simulink model "SMC"  (R2023a)
settings: Solver=FixedStepAuto  StartTime=0.0  StopTime=inf  RelTol=1e-3
undefined symbols (not defined in the file or in its folder): angular, linear
libraries: ros2lib x13

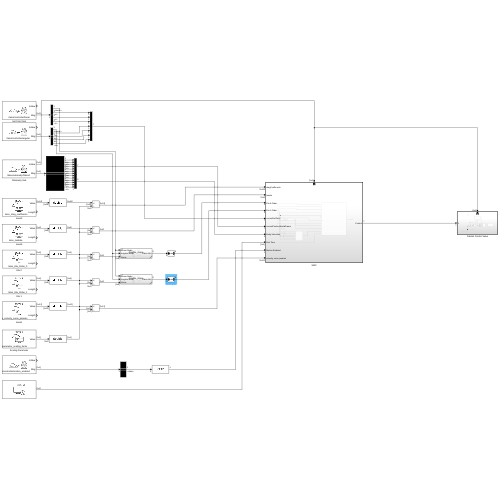
[thumbnail: Simulink's stored preview of the top-level diagram]
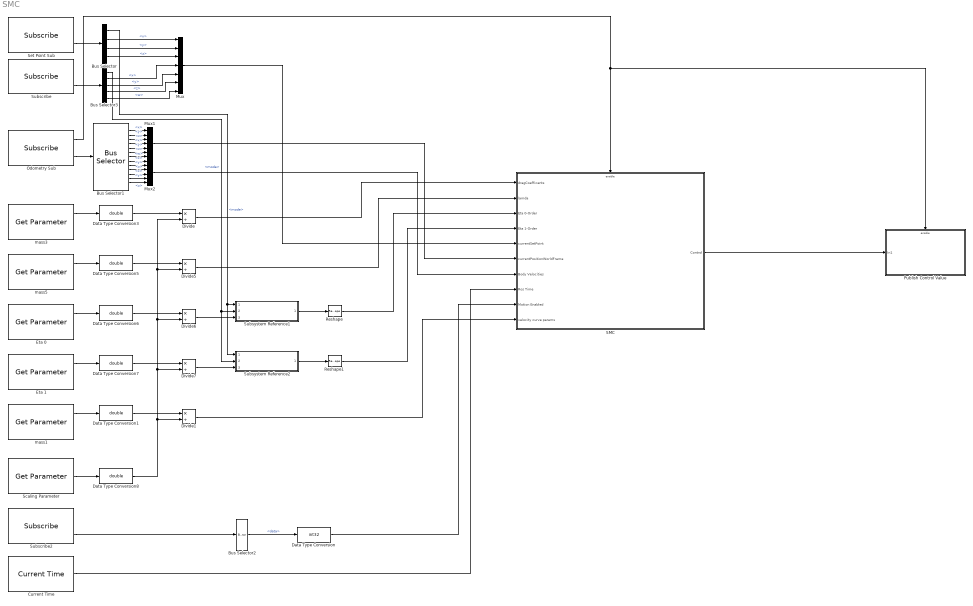
== system SMC ==
  Bus Selector : BusSelector  OutputSignals=mode,setpoint_vect.x,setpoint_vect.y,setpoint_vect.z
  Bus Selector1 : BusSelector  OutputSignals=pose.pose.position.x,pose.pose.position.y,pose.pose.position.z,pose.pose.orientation.x,pose.pose.orientation.y,pose.pose.orientation.z,pose.pose.orientation.w,twist.twist.linear.x,twist.twist.linear.y,twist.twist.linear.z,twist.twist.angular.x,twist.twist.angular.y,twist.twist.angular.z
  Bus Selector2 : BusSelector  OutputSignals=data
  Bus Selector3 : BusSelector  OutputSignals=mode,setpoint_quat.x,setpoint_quat.y,setpoint_quat.z,setpoint_quat.w
  Current Time : ros2lib/Current Time  OutputFormat=double  SampleTime=-1  ModelName=SMC
  Data Type Conversion : DataTypeConversion  OutDataTypeStr=int32  SaturateOnIntegerOverflow=off  RndMeth=Floor
  Data Type Conversion{1,3,5..8} (6 alike) : DataTypeConversion  OutDataTypeStr=double  SaturateOnIntegerOverflow=off  RndMeth=Floor
  Divide{,1,5..7} (5 alike) : Product  Inputs=*/
  Eta 0 : ros2lib/Get Parameter  ParameterName=talos_Eta_Order_0  ParameterType=int64[]  ParameterMaxArrayLength=6  ParameterInitialValue=0.0  SampleTime=-1  ModelName=SMC  BlockId=ParamGet_SMC_204
  Eta 1 : ros2lib/Get Parameter  ParameterName=talos_Eta_Order_1  ParameterType=int64[]  ParameterMaxArrayLength=6  ParameterInitialValue=0.0  SampleTime=-1  ModelName=SMC  BlockId=ParamGet_SMC_206
  Mux : Mux  Inputs=7
  Mux1 : Mux  Inputs=7
  Mux2 : Mux  Inputs=6
  Odometry Sub : ros2lib/Subscribe  topicSource=Specify your own  topic=/talos/odometry/filtered  messageType=nav_msgs/Odometry  sampleTime=0.01  QOSHistory=Keep last  QOSDepth=1  QOSReliability=Reliable  QOSDurability=Volatile
  Publish Control Value : Subsystem
  Reshape : Reshape  OutputDimensionality=Row vector (2-D)
  Reshape1 : Reshape  OutputDimensionality=Row vector (2-D)
  SMC : Subsystem
  Scaling Parameter : ros2lib/Get Parameter  ParameterName=parameter_scaling_factor  ParameterType=int64  ParameterMaxArrayLength=16  ParameterInitialValue=1000000  SampleTime=-1  ModelName=SMC  BlockId=ParamGet_SMC_208
  Set Point Sub : ros2lib/Subscribe  topicSource=Specify your own  topic=/talos/controller/linear  messageType=riptide_msgs2/ControllerCommand  sampleTime=0.01  QOSHistory=Keep last  QOSDepth=1  QOSReliability=Reliable  QOSDurability=Volatile
  Subscribe : ros2lib/Subscribe  topicSource=Specify your own  topic=/talos/controller/angular  messageType=riptide_msgs2/ControllerCommand  sampleTime=0.01  QOSHistory=Keep last  QOSDepth=1  QOSReliability=Reliable  QOSDurability=Volatile
  Subscribe2 : ros2lib/Subscribe  topicSource=Specify your own  topic=/talos/controller/motion_enabled  messageType=std_msgs/Bool  sampleTime=-1  QOSHistory=Keep last  QOSDepth=1  QOSReliability=Reliable  QOSDurability=Volatile
  Subsystem Reference1 : Subsystem  ReferencedSubsystem=Disable_Gains
  Subsystem Reference2 : Subsystem  ReferencedSubsystem=Disable_Gains
  mass1 : ros2lib/Get Parameter  ParameterName=talos_velocity_curve_params  ParameterType=int64[]  ParameterMaxArrayLength=12  ParameterInitialValue=[0,0,0,0,0,0,0,0,0,0,0,0]  SampleTime=-1  ModelName=SMC  BlockId=ParamGet_SMC_710
  mass3 : ros2lib/Get Parameter  ParameterName=talos_drag_coefficents  ParameterType=int64[]  ParameterMaxArrayLength=24  ParameterInitialValue=0.0  SampleTime=-1  ModelName=SMC  BlockId=ParamGet_SMC_197
  mass5 : ros2lib/Get Parameter  ParameterName=talos_lambda  ParameterType=int64[]  ParameterMaxArrayLength=6  ParameterInitialValue=0.0  SampleTime=-1  ModelName=SMC  BlockId=ParamGet_SMC_202
  wires:
  Mux/1 -> SMC/5(currentSetPoint)
  Odometry Sub/2 -> Bus Selector1/1
  Bus Selector1/1 -> Mux1/1  "<x>"
  Bus Selector1/2 -> Mux1/2  "<y>"
  Bus Selector1/3 -> Mux1/3  "<z>"
  Bus Selector1/4 -> Mux1/4  "<x>"
  Bus Selector1/5 -> Mux1/5  "<y>"
  Bus Selector1/6 -> Mux1/6  "<z>"
  Bus Selector1/7 -> Mux1/7  "<w>"
  Bus Selector1/8 -> Mux2/1  "<x>"
  Bus Selector1/9 -> Mux2/2  "<y>"
  Bus Selector1/10 -> Mux2/3  "<z>"
  Bus Selector1/11 -> Mux2/4  "<x>"
  Bus Selector1/12 -> Mux2/5  "<y>"
  Bus Selector1/13 -> Mux2/6  "<z>"
  Mux1/1 -> SMC/6(currentPositionWorldFrame)
  Mux2/1 -> SMC/7(Body Velocities)
  mass3/1 -> Data Type Conversion3/1
  mass5/1 -> Data Type Conversion5/1
  Eta 0/1 -> Data Type Conversion6/1
  Eta 1/1 -> Data Type Conversion7/1
  Scaling Parameter/1 -> Data Type Conversion8/1
  Data Type Conversion3/1 -> Divide/1
  Data Type Conversion5/1 -> Divide5/1
  Data Type Conversion6/1 -> Divide6/1
  Data Type Conversion7/1 -> Divide7/1
  Data Type Conversion8/1 -> Divide1/2, Divide7/2, Divide6/2, Divide/2, Divide5/2
  Divide/1 -> SMC/1(dragCoefficents)
  SMC/1(Control) -> Publish Control Value/1(In1)
  Odometry Sub/1 -> Publish Control Value/Enable, SMC/Enable
  Current Time/1 -> SMC/8(Ros Time)
  Subscribe2/2 -> Bus Selector2/1
  Bus Selector2/1 -> Data Type Conversion/1  "<data>"
  Data Type Conversion/1 -> SMC/9(Motion Enabled)
  mass1/1 -> Data Type Conversion1/1
  Data Type Conversion1/1 -> Divide1/1
  Divide1/1 -> SMC/10(velocity curve params)
  Set Point Sub/2 -> Bus Selector/1
  Bus Selector/2 -> Mux/1  "<x>"
  Bus Selector/3 -> Mux/2  "<y>"
  Bus Selector/4 -> Mux/3  "<z>"
  Subscribe/2 -> Bus Selector3/1
  Bus Selector3/2 -> Mux/4  "<x>"
  Bus Selector3/3 -> Mux/5  "<y>"
  Bus Selector3/4 -> Mux/6  "<z>"
  Bus Selector3/5 -> Mux/7  "<w>"
  Divide5/1 -> SMC/2(lamda)
  Divide6/1 -> Subsystem Reference1/3
  Subsystem Reference1/1 -> Reshape/1
  Divide7/1 -> Subsystem Reference2/3
  Subsystem Reference2/1 -> Reshape1/1
  Bus Selector/1 -> Subsystem Reference1/1, Subsystem Reference2/1  "<mode>"
  Bus Selector3/1 -> Subsystem Reference1/2, Subsystem Reference2/2  "<mode>"
  Reshape/1 -> SMC/3(Eta 0-Order)
  Reshape1/1 -> SMC/4(Eta 1-Order)

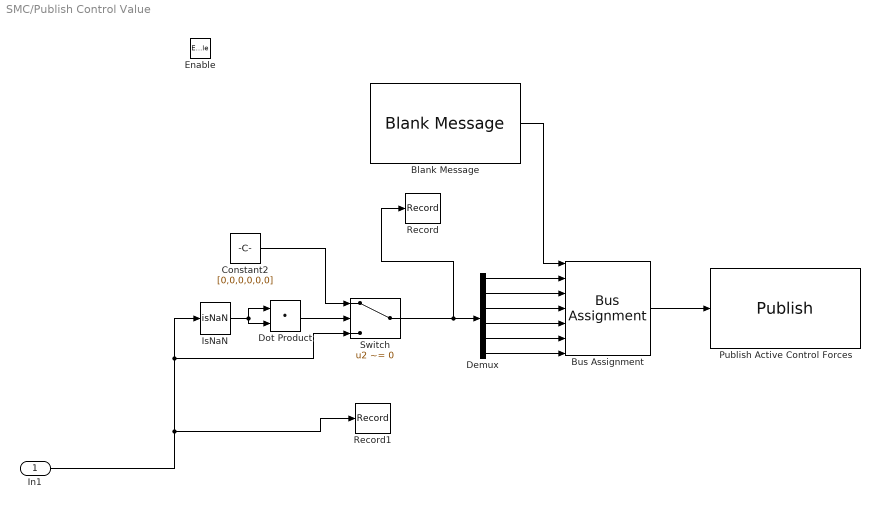
== system SMC/Publish Control Value ==
  In1 : Inport
  Enable : EnablePort
  Blank Message : ros2lib/Blank Message  messageClass=Message  entityType=geometry_msgs/Twist  messageType=geometry_msgs/Twist  SampleTime=inf
  Bus Assignment : BusAssignment  AssignedSignals=linear.x,linear.y,linear.z,angular.x,angular.y,angular.z
  Constant2 : Constant  Value=[0,0,0,0,0,0]
  Demux : Demux  Outputs=6
  Dot Product : DotProduct  OutDataTypeStr=Inherit: Inherit via internal rule
  IsNaN : RelationalOperator  Operator=isNaN  OutDataTypeStr=boolean  RndMeth=Simplest  InputSameDT=off
  Publish Active Control Forces : ros2lib/Publish  topicSource=Specify your own  topic=/talos/controller/active_body_force/smc  messageType=geometry_msgs/Twist  QOSHistory=Keep last  QOSDepth=1  QOSReliability=Reliable  QOSDurability=Volatile
  Record : Record  FileSettingsInternal="{\"entries\":[{\"content\":{\"excelSettings\":{\"content\":{},\"type\":\"Streamout.ExcelSettings\"}},\"type\":\"Streamout.FileSettingStorage\",\"uuid\":\"\"}],\"packageUris\":[\"http:\\/\\/schema.mathworks.com\\/mf0\\/streamout_blocks\\/R2020a\"],\"version\":\"1.0\"}"  Layout=[1 1]  SignalsInternal="{\"entries\":[{\"content\":{\"signals\":[{\"content\":{\"blockPath\":[],\"dimensions\":[6],\"domain\":\"\",\"hasChildren\":true,\"lineColor\":\"#77ac30\",\"port\":1,\"signalID\":4244,\"signalName\":\"Switch\"},\"type\":\"RecordBlkView.Signal\",\"uuid\":\"\"},{\"content\":{\"blockPath\":[],\"channel\":[1],\"dimensions\":[6],\"domain\":\"\",\"lineColor\":\"#77ac30\",\"parentID\":4244,\"port\":1,\"signalID\":4245,\"signalName\":\"Switch\"},\"type\":\"RecordBlkView.S ...(+1160 chars)"  VisualizationBindings="{\"sparklinesplugin\":{\"info\":[{\"bindingParametersList\":[],\"subplotID\":1}]}}"
  Record1 : Record  FileSettingsInternal="{\"entries\":[{\"content\":{\"excelSettings\":{\"content\":{},\"type\":\"Streamout.ExcelSettings\"}},\"type\":\"Streamout.FileSettingStorage\",\"uuid\":\"\"}],\"packageUris\":[\"http:\\/\\/schema.mathworks.com\\/mf0\\/streamout_blocks\\/R2020a\"],\"version\":\"1.0\"}"  Layout=[1 1]  SignalsInternal="{\"entries\":[{\"content\":{\"signals\":[{\"content\":{\"blockPath\":[],\"dimensions\":[6],\"domain\":\"\",\"hasChildren\":true,\"lineColor\":\"#a2142f\",\"port\":1,\"signalID\":4210,\"signalName\":\"In1\"},\"type\":\"RecordBlkView.Signal\",\"uuid\":\"\"},{\"content\":{\"blockPath\":[],\"channel\":[1],\"dimensions\":[6],\"domain\":\"\",\"lineColor\":\"#22b573\",\"parentID\":4210,\"plots\":[1],\"port\":1,\"signalID\":4211,\"signalName\":\"In1\"},\"type\":\"RecordBlk ...(+1199 chars)"  VisualizationBindings="{\"sparklinesplugin\":{\"info\":[{\"bindingParametersList\":[],\"subplotID\":1}]}}"
  Switch : Switch  Criteria=u2 ~= 0  SaturateOnIntegerOverflow=off  InputSameDT=off
  wires:
  Blank Message/1 -> Bus Assignment/1
  Switch/1 -> Record/1, Demux/1
  IsNaN/1 -> Dot Product/1, Dot Product/2
  Constant2/1 -> Switch/1
  Dot Product/1 -> Switch/2
  Demux/1 -> Bus Assignment/2
  Demux/2 -> Bus Assignment/3
  Demux/6 -> Bus Assignment/7
  Demux/3 -> Bus Assignment/4
  Demux/5 -> Bus Assignment/6
  In1/1 -> Record1/1, IsNaN/1, Switch/3
  Demux/4 -> Bus Assignment/5
  Bus Assignment/1 -> Publish Active Control Forces/1

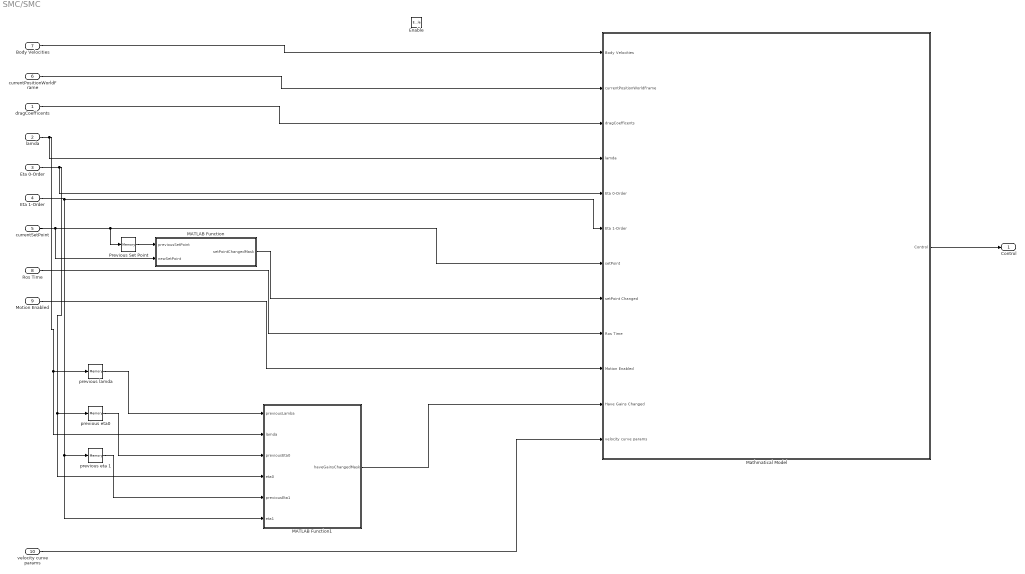
== system SMC/SMC ==
  dragCoefficents : Inport
  lamda : Inport  Port=2
  Eta 0-Order : Inport  Port=3
  Eta 1-Order : Inport  Port=4
  currentSetPoint : Inport  Port=5
  currentPositionWorldFrame : Inport  Port=6
  Body Velocities : Inport  Port=7
  Ros Time : Inport  Port=8
  Motion Enabled : Inport  Port=9
  velocity curve params : Inport  Port=10
  Enable : EnablePort
  MATLAB Function : MATLAB Function  TreatAsAtomicUnit=on
  MATLAB Function1 : MATLAB Function  TreatAsAtomicUnit=on
  Mathmatical Model : Subsystem
  Previous Set Point : Memory  InitialCondition=[0,0,0,0,0,0,0]  InheritSampleTime=on
  previous eta 1 : Memory  InheritSampleTime=on
  previous eta0 : Memory  InheritSampleTime=on
  previous lamda : Memory  InheritSampleTime=on
  Control : Outport
  wires:
  dragCoefficents/1 -> Mathmatical Model/3(dragCoefficents)
  Mathmatical Model/1(Control) -> Control/1
  currentSetPoint/1 -> MATLAB Function/2(newSetPoint), Previous Set Point/1, Mathmatical Model/7(setPoint)
  currentPositionWorldFrame/1 -> Mathmatical Model/2(currentPositionWorldFrame)
  Body Velocities/1 -> Mathmatical Model/1(Body Velocities)
  MATLAB Function/1(setPointChangedMask) -> Mathmatical Model/8(setPoint Changed)
  Previous Set Point/1 -> MATLAB Function/1(previousSetPoint)
  Ros Time/1 -> Mathmatical Model/9(Ros Time)
  Motion Enabled/1 -> Mathmatical Model/10(Motion Enabled)
  previous lamda/1 -> MATLAB Function1/1(previousLamba)
  previous eta0/1 -> MATLAB Function1/3(previousEta0)
  previous eta 1/1 -> MATLAB Function1/5(previousEta1)
  lamda/1 -> Mathmatical Model/4(lamda), MATLAB Function1/2(lamda), previous lamda/1
  Eta 0-Order/1 -> Mathmatical Model/5(Eta 0-Order), previous eta0/1, MATLAB Function1/4(eta0)
  Eta 1-Order/1 -> previous eta 1/1, MATLAB Function1/6(eta1), Mathmatical Model/6(Eta 1-Order)
  MATLAB Function1/1(haveGainsChangedMask) -> Mathmatical Model/11(Have Gains Changed)
  velocity curve params/1 -> Mathmatical Model/12(velocity curve params)

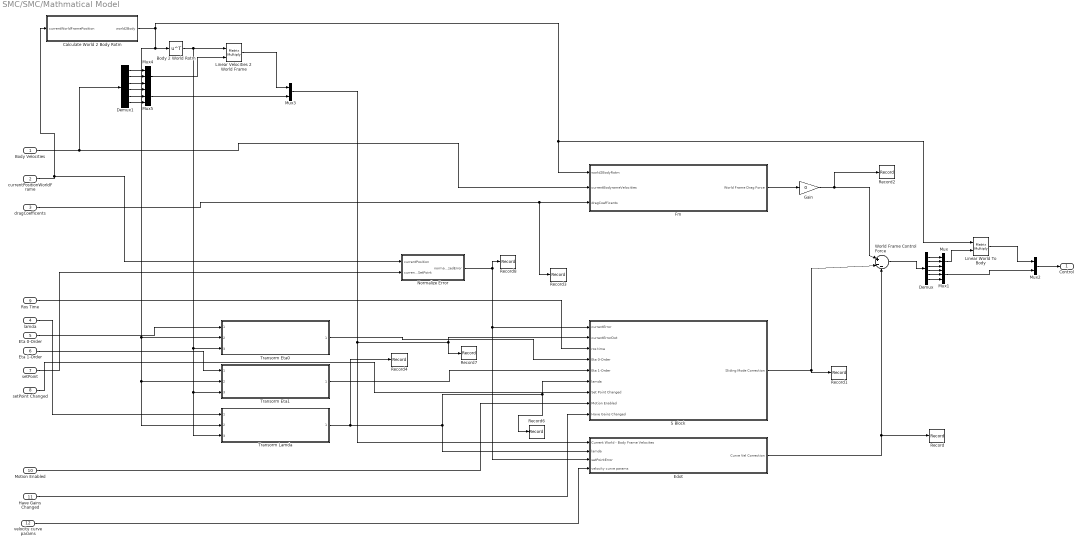
== system SMC/SMC/Mathmatical Model ==
  Body Velocities : Inport
  currentPositionWorldFrame : Inport  Port=2
  dragCoefficents : Inport  Port=3
  lamda : Inport  Port=4
  Eta 0-Order : Inport  Port=5
  Eta 1-Order : Inport  Port=6
  setPoint : Inport  Port=7
  setPoint Changed : Inport  Port=8
  Ros Time : Inport  Port=9
  Motion Enabled : Inport  Port=10
  Have Gains Changed : Inport  Port=11
  velocity curve params : Inport  Port=12
  Body 2 World Rotm : Math  Operator=transpose
  Calculate World 2 Body Rotm : MATLAB Function  TreatAsAtomicUnit=on
  Demux : Demux  Outputs=6
  Demux1 : Demux  Outputs=6
  Edot : Subsystem
  Fm : Subsystem
  Gain : Gain  Gain=0
  Linear Velocities 2 World Frame : Product  Multiplication=Matrix(*)
  Linear World To Body : Product  Multiplication=Matrix(*)
  Mux{,1,4..5} (4 alike) : Mux  Inputs=3
  Mux2 : Mux  Inputs=2
  Mux3 : Mux  Inputs=2
  Normalize Error : MATLAB Function  TreatAsAtomicUnit=on
  Record : Record  FileSettingsInternal="{\"entries\":[{\"content\":{\"excelSettings\":{\"content\":{},\"type\":\"Streamout.ExcelSettings\"}},\"type\":\"Streamout.FileSettingStorage\",\"uuid\":\"\"}],\"packageUris\":[\"http:\\/\\/schema.mathworks.com\\/mf0\\/streamout_blocks\\/R2020a\"],\"version\":\"1.0\"}"  Layout=[1 1]  SignalsInternal="{\"entries\":[{\"content\":{\"signals\":[{\"content\":{\"blockPath\":[],\"dimensions\":[6,1],\"domain\":\"\",\"hasChildren\":true,\"lineColor\":\"#ff13a6\",\"port\":1,\"signalID\":4045,\"signalName\":\"Edot\"},\"type\":\"RecordBlkView.Signal\",\"uuid\":\"\"},{\"content\":{\"blockPath\":[],\"channel\":[1,1],\"dimensions\":[6,1],\"domain\":\"\",\"lineColor\":\"#4dbeee\",\"parentID\":4045,\"port\":1,\"signalID\":4046,\"signalName\":\"Edot\"},\"type\":\"RecordBlkView ...(+1172 chars)"  VisualizationBindings="{\"sparklinesplugin\":{\"info\":[{\"bindingParametersList\":[],\"subplotID\":1}]}}"
  Record1 : Record  FileSettingsInternal="{\"entries\":[{\"content\":{\"excelSettings\":{\"content\":{},\"type\":\"Streamout.ExcelSettings\"}},\"type\":\"Streamout.FileSettingStorage\",\"uuid\":\"\"}],\"packageUris\":[\"http:\\/\\/schema.mathworks.com\\/mf0\\/streamout_blocks\\/R2020a\"],\"version\":\"1.0\"}"  Layout=[1 1]  SignalsInternal="{\"entries\":[{\"content\":{\"signals\":[{\"content\":{\"blockPath\":[],\"dimensions\":[6,1],\"domain\":\"\",\"hasChildren\":true,\"lineColor\":\"#22b573\",\"port\":1,\"signalID\":4227,\"signalName\":\"S Block\"},\"type\":\"RecordBlkView.Signal\",\"uuid\":\"\"},{\"content\":{\"blockPath\":[],\"channel\":[1,1],\"dimensions\":[6,1],\"domain\":\"\",\"lineColor\":\"#0072bd\",\"parentID\":4227,\"port\":1,\"signalID\":4228,\"signalName\":\"S Block\"},\"type\":\"RecordB ...(+1193 chars)"  VisualizationBindings="{\"sparklinesplugin\":{\"info\":[{\"bindingParametersList\":[],\"subplotID\":1}]}}"
  Record2 : Record  FileSettingsInternal="{\"entries\":[{\"content\":{\"excelSettings\":{\"content\":{},\"type\":\"Streamout.ExcelSettings\"}},\"type\":\"Streamout.FileSettingStorage\",\"uuid\":\"\"}],\"packageUris\":[\"http:\\/\\/schema.mathworks.com\\/mf0\\/streamout_blocks\\/R2020a\"],\"version\":\"1.0\"}"  Layout=[1 1]  SignalsInternal="{\"entries\":[{\"content\":{\"signals\":[{\"content\":{\"blockPath\":[],\"dimensions\":[6],\"domain\":\"\",\"hasChildren\":true,\"lineColor\":\"#d95319\",\"port\":1,\"signalID\":3994,\"signalName\":\"Gain\"},\"type\":\"RecordBlkView.Signal\",\"uuid\":\"\"},{\"content\":{\"blockPath\":[],\"channel\":[1],\"dimensions\":[6],\"domain\":\"\",\"lineColor\":\"#edb120\",\"parentID\":3994,\"plots\":[1],\"port\":1,\"signalID\":3995,\"signalName\":\"Gain\"},\"type\":\"RecordB ...(+1206 chars)"  VisualizationBindings="{\"sparklinesplugin\":{\"info\":[{\"bindingParametersList\":[],\"subplotID\":1}]}}"
  Record3 : Record  FileSettingsInternal="{\"entries\":[{\"content\":{\"excelSettings\":{\"content\":{},\"type\":\"Streamout.ExcelSettings\"}},\"type\":\"Streamout.FileSettingStorage\",\"uuid\":\"\"}],\"packageUris\":[\"http:\\/\\/schema.mathworks.com\\/mf0\\/streamout_blocks\\/R2020a\"],\"version\":\"1.0\"}"  Layout=[1 1]  SignalsInternal="{\"entries\":[{\"content\":{\"signals\":[{\"content\":{\"blockPath\":[],\"dimensions\":[1,24],\"domain\":\"\",\"hasChildren\":true,\"lineColor\":\"#7e2f8e\",\"port\":1,\"signalID\":3941,\"signalName\":\"dragCoefficents\"},\"type\":\"RecordBlkView.Signal\",\"uuid\":\"\"},{\"content\":{\"blockPath\":[],\"channel\":[1,1],\"dimensions\":[1,24],\"domain\":\"\",\"lineColor\":\"#77ac30\",\"parentID\":3941,\"plots\":[1],\"port\":1,\"signalID\":3942,\"signalName\":\"dra ...(+5141 chars)"  VisualizationBindings="{\"sparklinesplugin\":{\"info\":[{\"bindingParametersList\":[],\"subplotID\":1}]}}"
  Record4 : Record  FileSettingsInternal="{\"entries\":[{\"content\":{\"excelSettings\":{\"content\":{},\"type\":\"Streamout.ExcelSettings\"}},\"type\":\"Streamout.FileSettingStorage\",\"uuid\":\"\"}],\"packageUris\":[\"http:\\/\\/schema.mathworks.com\\/mf0\\/streamout_blocks\\/R2020a\"],\"version\":\"1.0\"}"  Layout=[1 1]  SignalsInternal="{\"entries\":[{\"content\":{\"signals\":[{\"content\":{\"blockPath\":[],\"dimensions\":[6],\"domain\":\"\",\"hasChildren\":true,\"lineColor\":\"#4dbeee\",\"port\":1,\"signalID\":3907,\"signalName\":\"Transorm Lamda\"},\"type\":\"RecordBlkView.Signal\",\"uuid\":\"\"},{\"content\":{\"blockPath\":[],\"channel\":[1],\"dimensions\":[6],\"domain\":\"\",\"lineColor\":\"#64d413\",\"parentID\":3907,\"plots\":[1],\"port\":1,\"signalID\":3908,\"signalName\":\"Transorm Lam ...(+1276 chars)"  VisualizationBindings="{\"sparklinesplugin\":{\"info\":[{\"bindingParametersList\":[],\"subplotID\":1}]}}"
  Record6 : Record  FileSettingsInternal="{\"entries\":[{\"content\":{\"excelSettings\":{\"content\":{},\"type\":\"Streamout.ExcelSettings\"}},\"type\":\"Streamout.FileSettingStorage\",\"uuid\":\"\"}],\"packageUris\":[\"http:\\/\\/schema.mathworks.com\\/mf0\\/streamout_blocks\\/R2020a\"],\"version\":\"1.0\"}"  Layout=[1 1]  SignalsInternal="{\"entries\":[{\"content\":{\"signals\":[{\"content\":{\"blockPath\":[],\"dimensions\":[6],\"domain\":\"\",\"hasChildren\":true,\"lineColor\":\"#139fff\",\"port\":1,\"signalID\":3924,\"signalName\":\"Transorm Lamda\"},\"type\":\"RecordBlkView.Signal\",\"uuid\":\"\"},{\"content\":{\"blockPath\":[],\"channel\":[1],\"dimensions\":[6],\"domain\":\"\",\"lineColor\":\"#64d413\",\"parentID\":3924,\"plots\":[1],\"port\":1,\"signalID\":3925,\"signalName\":\"Transorm Lam ...(+1240 chars)"  VisualizationBindings="{\"sparklinesplugin\":{\"info\":[{\"bindingParametersList\":[],\"subplotID\":1}]}}"
  Record7 : Record  FileSettingsInternal="{\"entries\":[{\"content\":{\"excelSettings\":{\"content\":{},\"type\":\"Streamout.ExcelSettings\"}},\"type\":\"Streamout.FileSettingStorage\",\"uuid\":\"\"}],\"packageUris\":[\"http:\\/\\/schema.mathworks.com\\/mf0\\/streamout_blocks\\/R2020a\"],\"version\":\"1.0\"}"  Layout=[1 1]  SignalsInternal="{\"entries\":[{\"content\":{\"signals\":[{\"content\":{\"blockPath\":[],\"dimensions\":[6],\"domain\":\"\",\"hasChildren\":true,\"lineColor\":\"#b746ff\",\"port\":1,\"signalID\":4011,\"signalName\":\"Mux3\"},\"type\":\"RecordBlkView.Signal\",\"uuid\":\"\"},{\"content\":{\"blockPath\":[],\"channel\":[1],\"dimensions\":[6],\"domain\":\"\",\"lineColor\":\"#edb120\",\"parentID\":4011,\"plots\":[1],\"port\":1,\"signalID\":4012,\"signalName\":\"Mux3\"},\"type\":\"RecordB ...(+1170 chars)"  VisualizationBindings="{\"sparklinesplugin\":{\"info\":[{\"bindingParametersList\":[],\"subplotID\":1}]}}"
  Record8 : Record  FileSettingsInternal="{\"entries\":[{\"content\":{\"excelSettings\":{\"content\":{},\"type\":\"Streamout.ExcelSettings\"}},\"type\":\"Streamout.FileSettingStorage\",\"uuid\":\"\"}],\"packageUris\":[\"http:\\/\\/schema.mathworks.com\\/mf0\\/streamout_blocks\\/R2020a\"],\"version\":\"1.0\"}"  Layout=[1 1]  SignalsInternal="{\"entries\":[{\"content\":{\"signals\":[{\"content\":{\"blockPath\":[],\"dimensions\":[1,6],\"domain\":\"\",\"hasChildren\":true,\"lineColor\":\"#ff13a6\",\"port\":1,\"signalID\":4028,\"signalName\":\"Normalize Error\"},\"type\":\"RecordBlkView.Signal\",\"uuid\":\"\"},{\"content\":{\"blockPath\":[],\"channel\":[1,1],\"dimensions\":[1,6],\"domain\":\"\",\"lineColor\":\"#a2142f\",\"parentID\":4028,\"plots\":[1],\"port\":1,\"signalID\":4029,\"signalName\":\"Norma ...(+1273 chars)"  VisualizationBindings="{\"sparklinesplugin\":{\"info\":[{\"bindingParametersList\":[],\"subplotID\":1}]}}"
  S Block : Subsystem
  Transorm Eta0 : Subsystem  ReferencedSubsystem=Tranfsform_Linear_Gains_To_World
  Transorm Eta1 : Subsystem  ReferencedSubsystem=Tranfsform_Linear_Gains_To_World
  Transorm Lamda : Subsystem  ReferencedSubsystem=Tranfsform_Linear_Gains_To_World
  World Frame Control Force : Sum  Inputs=|+--
  Control : Outport
  wires:
  Body Velocities/1 -> Fm/2(currentBodyrameVelocities), Demux1/1
  currentPositionWorldFrame/1 -> Normalize Error/1(currentPosition), Calculate World 2 Body Rotm/1(currentWorldFramePosition)
  S Block/1("Sliding Mode Correction ") -> World Frame Control Force/2, Record1/1
  World Frame Control Force/1 -> Demux/1
  Demux/1 -> Mux/1
  Demux/2 -> Mux/2
  Demux/3 -> Mux/3
  Demux/6 -> Mux1/3
  Demux/5 -> Mux1/2
  Demux/4 -> Mux1/1
  Mux/1 -> Linear World To Body/2
  Linear World To Body/1 -> Mux2/1
  Mux1/1 -> Mux2/2
  Mux2/1 -> Control/1
  Calculate World 2 Body Rotm/1(world2Body) -> Body 2 World Rotm/1, Transorm Eta0/2, Transorm Eta1/2, Transorm Lamda/2, Linear World To Body/1, Fm/1(world2BodyRotm)
  dragCoefficents/1 -> Record3/1, Fm/3(dragCoefficents)
  Linear Velocities 2 World Frame/1 -> Mux3/1
  Mux4/1 -> Linear Velocities 2 World Frame/2
  Demux1/2 -> Mux4/2
  Demux1/1 -> Mux4/1
  Demux1/3 -> Mux4/3
  Demux1/5 -> Mux5/2
  Demux1/4 -> Mux5/1
  Demux1/6 -> Mux5/3
  Fm/1(World Frame Drag Force) -> Gain/1
  Mux5/1 -> Mux3/2
  Transorm Lamda/1 -> Record4/1, Record6/1, S Block/6(lamda), Edot/2(lamda)
  Transorm Eta1/1 -> S Block/5(Eta 1-Order)
  lamda/1 -> Transorm Lamda/1
  Eta 0-Order/1 -> Transorm Eta0/1
  Mux3/1 -> Record7/1, S Block/2(currentErrorDot), Edot/1(Current World - Body Frame Velocites)
  setPoint Changed/1 -> S Block/7(Set Point Changed)
  Ros Time/1 -> S Block/3(ros time)
  Normalize Error/1(normalizedError) -> Record8/1, Edot/3(setPointError), S Block/1(currentError)
  setPoint/1 -> Normalize Error/2(currentSetPoint)
  Eta 1-Order/1 -> Transorm Eta1/1
  Gain/1 -> Record2/1, World Frame Control Force/1
  Edot/1(Curve Vel Correction) -> Record/1, World Frame Control Force/3
  Body 2 World Rotm/1 -> Transorm Eta0/3, Transorm Eta1/3, Transorm Lamda/3, Linear Velocities 2 World Frame/1
  Transorm Eta0/1 -> S Block/4(Eta 0-Order)
  Motion Enabled/1 -> S Block/8(Motion Enabled)
  Have Gains Changed/1 -> S Block/9(Have Gains Changed)
  velocity curve params/1 -> Edot/4(velocity curve params)

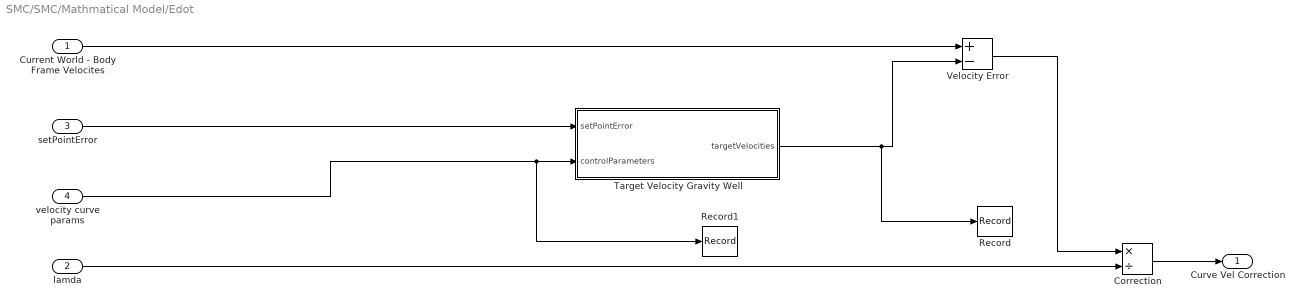
== system SMC/SMC/Mathmatical Model/Edot ==
  Current World - Body Frame Velocites : Inport
  lamda : Inport  Port=2
  setPointError : Inport  Port=3
  velocity curve params : Inport  Port=4
  Correction : Product  Inputs=*/
  Record : Record  FileSettingsInternal="{\"entries\":[{\"content\":{\"excelSettings\":{\"content\":{},\"type\":\"Streamout.ExcelSettings\"}},\"type\":\"Streamout.FileSettingStorage\",\"uuid\":\"\"}],\"packageUris\":[\"http:\\/\\/schema.mathworks.com\\/mf0\\/streamout_blocks\\/R2020a\"],\"version\":\"1.0\"}"  Layout=[1 1]  SignalsInternal="{\"entries\":[{\"content\":{\"signals\":[{\"content\":{\"blockPath\":[],\"dimensions\":[6,1],\"domain\":\"\",\"hasChildren\":true,\"lineColor\":\"#22b573\",\"port\":1,\"signalID\":4153,\"signalName\":\"Target Velocity Gravity Well\"},\"type\":\"RecordBlkView.Signal\",\"uuid\":\"\"},{\"content\":{\"blockPath\":[],\"channel\":[1,1],\"dimensions\":[6,1],\"domain\":\"\",\"lineColor\":\"#d95319\",\"parentID\":4153,\"plots\":[1],\"port\":1,\"signalID\":4154,\"signa ...(+1340 chars)"  VisualizationBindings="{\"sparklinesplugin\":{\"info\":[{\"bindingParametersList\":[],\"subplotID\":1}]}}"
  Record1 : Record  FileSettingsInternal="{\"entries\":[{\"content\":{\"excelSettings\":{\"content\":{},\"type\":\"Streamout.ExcelSettings\"}},\"type\":\"Streamout.FileSettingStorage\",\"uuid\":\"\"}],\"packageUris\":[\"http:\\/\\/schema.mathworks.com\\/mf0\\/streamout_blocks\\/R2020a\"],\"version\":\"1.0\"}"  Layout=[1 1]  SignalsInternal="{\"entries\":[{\"content\":{\"signals\":[{\"content\":{\"blockPath\":[],\"dimensions\":[1,12],\"domain\":\"\",\"hasChildren\":true,\"lineColor\":\"#d95319\",\"port\":1,\"signalID\":4170,\"signalName\":\"velocity curve params\"},\"type\":\"RecordBlkView.Signal\",\"uuid\":\"\"},{\"content\":{\"blockPath\":[],\"channel\":[1,1],\"dimensions\":[1,12],\"domain\":\"\",\"lineColor\":\"#edb120\",\"parentID\":4170,\"plots\":[1],\"port\":1,\"signalID\":4171,\"signalName ...(+2639 chars)"  VisualizationBindings="{\"sparklinesplugin\":{\"info\":[{\"bindingParametersList\":[],\"subplotID\":1}]}}"
  Target Velocity Gravity Well : MATLAB Function  TreatAsAtomicUnit=on
  Velocity Error : Sum  Inputs=+-
  Curve Vel Correction : Outport
  wires:
  Correction/1 -> Curve Vel Correction/1
  lamda/1 -> Correction/2
  Current World - Body Frame Velocites/1 -> Velocity Error/1
  Velocity Error/1 -> Correction/1
  setPointError/1 -> Target Velocity Gravity Well/1(setPointError)
  Target Velocity Gravity Well/1(targetVelocities) -> Record/1, Velocity Error/2
  velocity curve params/1 -> Record1/1, Target Velocity Gravity Well/2(controlParameters)

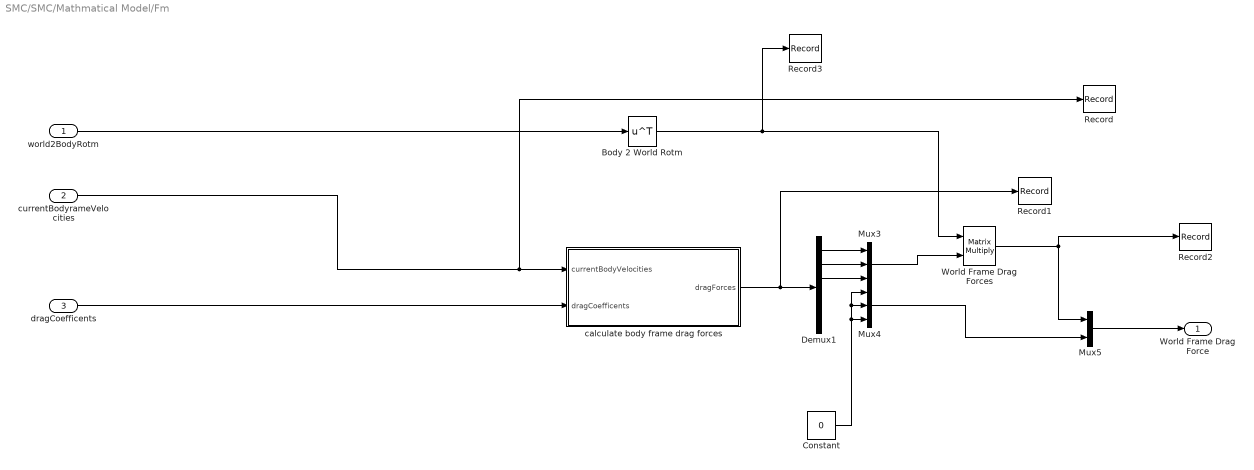
== system SMC/SMC/Mathmatical Model/Fm ==
  world2BodyRotm : Inport
  currentBodyrameVelocities : Inport  Port=2
  dragCoefficents : Inport  Port=3
  Body 2 World Rotm : Math  Operator=transpose
  Constant : Constant  Value=0
  Demux1 : Demux  Outputs=6
  Mux3 : Mux  Inputs=3
  Mux4 : Mux  Inputs=3
  Mux5 : Mux  Inputs=2
  Record : Record  FileSettingsInternal="{\"entries\":[{\"content\":{\"excelSettings\":{\"content\":{},\"type\":\"Streamout.ExcelSettings\"}},\"type\":\"Streamout.FileSettingStorage\",\"uuid\":\"\"}],\"packageUris\":[\"http:\\/\\/schema.mathworks.com\\/mf0\\/streamout_blocks\\/R2020a\"],\"version\":\"1.0\"}"  Layout=[1 1]  SignalsInternal="{\"entries\":[{\"content\":{\"signals\":[{\"content\":{\"blockPath\":[],\"dimensions\":[6],\"domain\":\"\",\"hasChildren\":true,\"lineColor\":\"#7e2f8e\",\"port\":1,\"signalID\":4119,\"signalName\":\"currentBodyrameVelocities\"},\"type\":\"RecordBlkView.Signal\",\"uuid\":\"\"},{\"content\":{\"blockPath\":[],\"channel\":[1],\"dimensions\":[6],\"domain\":\"\",\"lineColor\":\"#b746ff\",\"parentID\":4119,\"plots\":[1],\"port\":1,\"signalID\":4120,\"signalName\":\"c ...(+1341 chars)"  VisualizationBindings="{\"sparklinesplugin\":{\"info\":[{\"bindingParametersList\":[],\"subplotID\":1}]}}"
  Record1 : Record  FileSettingsInternal="{\"entries\":[{\"content\":{\"excelSettings\":{\"content\":{},\"type\":\"Streamout.ExcelSettings\"}},\"type\":\"Streamout.FileSettingStorage\",\"uuid\":\"\"}],\"packageUris\":[\"http:\\/\\/schema.mathworks.com\\/mf0\\/streamout_blocks\\/R2020a\"],\"version\":\"1.0\"}"  Layout=[1 1]  SignalsInternal="{\"entries\":[{\"content\":{\"signals\":[{\"content\":{\"blockPath\":[],\"dimensions\":[6,1],\"domain\":\"\",\"hasChildren\":true,\"lineColor\":\"#4dbeee\",\"port\":1,\"signalID\":4085,\"signalName\":\"calculate body frame drag forces\"},\"type\":\"RecordBlkView.Signal\",\"uuid\":\"\"},{\"content\":{\"blockPath\":[],\"channel\":[1,1],\"dimensions\":[6,1],\"domain\":\"\",\"lineColor\":\"#139fff\",\"parentID\":4085,\"plots\":[1],\"port\":1,\"signalID\":4086,\"s ...(+1428 chars)"  VisualizationBindings="{\"sparklinesplugin\":{\"info\":[{\"bindingParametersList\":[],\"subplotID\":1}]}}"
  Record2 : Record  FileSettingsInternal="{\"entries\":[{\"content\":{\"excelSettings\":{\"content\":{},\"type\":\"Streamout.ExcelSettings\"}},\"type\":\"Streamout.FileSettingStorage\",\"uuid\":\"\"}],\"packageUris\":[\"http:\\/\\/schema.mathworks.com\\/mf0\\/streamout_blocks\\/R2020a\"],\"version\":\"1.0\"}"  SignalsInternal="{\"entries\":[{\"content\":{\"signals\":[{\"content\":{\"blockPath\":[],\"dimensions\":[3],\"domain\":\"\",\"hasChildren\":true,\"lineColor\":\"#139fff\",\"port\":1,\"signalID\":4199,\"signalName\":\"World Frame Drag Forces\"},\"type\":\"RecordBlkView.Signal\",\"uuid\":\"\"},{\"content\":{\"blockPath\":[],\"channel\":[1],\"dimensions\":[3],\"domain\":\"\",\"lineColor\":\"#b746ff\",\"parentID\":4199,\"plots\":[1],\"port\":1,\"signalID\":4200,\"signalName\":\"Wor ...(+661 chars)"  VisualizationBindings="{\"sparklinesplugin\":{\"info\":[{\"bindingParametersList\":[],\"subplotID\":1}]}}"
  Record3 : Record  FileSettingsInternal="{\"entries\":[{\"content\":{\"excelSettings\":{\"content\":{},\"type\":\"Streamout.ExcelSettings\"}},\"type\":\"Streamout.FileSettingStorage\",\"uuid\":\"\"}],\"packageUris\":[\"http:\\/\\/schema.mathworks.com\\/mf0\\/streamout_blocks\\/R2020a\"],\"version\":\"1.0\"}"  Layout=[1 1]  SignalsInternal="{\"entries\":[{\"content\":{\"signals\":[{\"content\":{\"blockPath\":[],\"dimensions\":[3,3],\"domain\":\"\",\"hasChildren\":true,\"lineColor\":\"#b746ff\",\"port\":1,\"signalID\":4062,\"signalName\":\"Body 2 World Rotm\"},\"type\":\"RecordBlkView.Signal\",\"uuid\":\"\"},{\"content\":{\"blockPath\":[],\"channel\":[1,1],\"dimensions\":[3,3],\"domain\":\"\",\"lineColor\":\"#a2142f\",\"parentID\":4062,\"plots\":[1],\"port\":1,\"signalID\":4063,\"signalName\":\"Bod ...(+1995 chars)"  VisualizationBindings="{\"sparklinesplugin\":{\"info\":[{\"bindingParametersList\":[],\"subplotID\":1}]}}"
  World Frame Drag Forces : Product  Multiplication=Matrix(*)
  calculate body frame drag forces : MATLAB Function  TreatAsAtomicUnit=on
  World Frame Drag Force : Outport
  wires:
  World Frame Drag Forces/1 -> Mux5/1, Record2/1
  Demux1/1 -> Mux3/1
  Mux3/1 -> World Frame Drag Forces/2
  Demux1/3 -> Mux3/3
  Mux5/1 -> World Frame Drag Force/1
  Demux1/2 -> Mux3/2
  currentBodyrameVelocities/1 -> Record/1, calculate body frame drag forces/1(currentBodyVelocities)
  dragCoefficents/1 -> calculate body frame drag forces/2(dragCoefficents)
  world2BodyRotm/1 -> Body 2 World Rotm/1
  Body 2 World Rotm/1 -> Record3/1, World Frame Drag Forces/1
  calculate body frame drag forces/1(dragForces) -> Record1/1, Demux1/1
  Mux4/1 -> Mux5/2
  Constant/1 -> Mux4/3, Mux4/2, Mux4/1

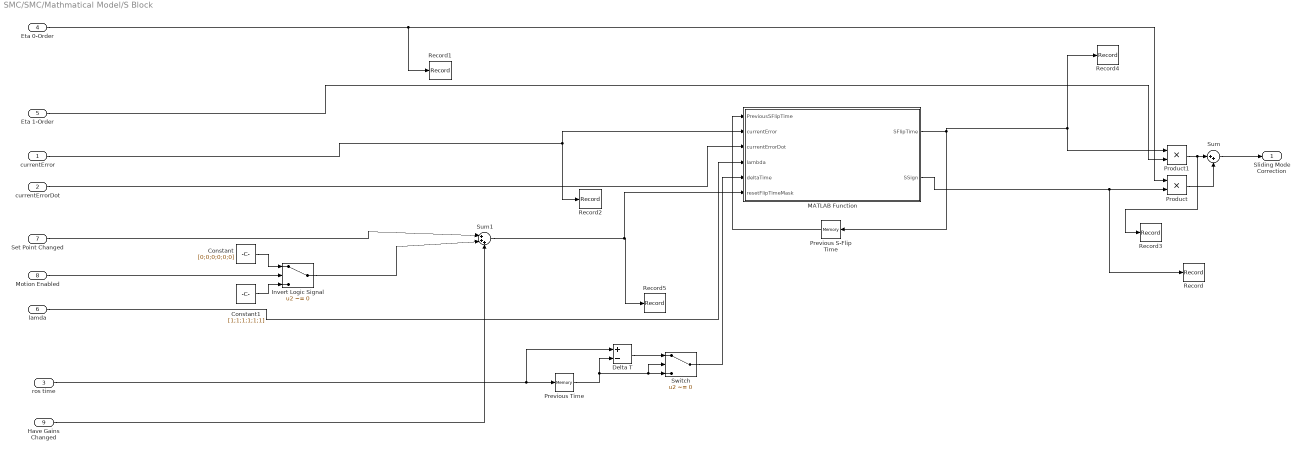
== system SMC/SMC/Mathmatical Model/S Block ==
  currentError : Inport
  currentErrorDot : Inport  Port=2
  ros time : Inport  Port=3
  Eta 0-Order : Inport  Port=4
  Eta 1-Order : Inport  Port=5
  lamda : Inport  Port=6
  Set Point Changed : Inport  Port=7
  Motion Enabled : Inport  Port=8
  Have Gains Changed : Inport  Port=9
  Constant : Constant  Value=[0;0;0;0;0;0]
  Constant1 : Constant  Value=[1;1;1;1;1;1]
  Delta T : Sum  Inputs=+-
  Invert Logic Signal : Switch  Criteria=u2 ~= 0  SaturateOnIntegerOverflow=off  InputSameDT=off
  MATLAB Function : MATLAB Function  TreatAsAtomicUnit=on
  Previous S-Flip Time : Memory  InitialCondition=[0;0;0;0;0;0]  InheritSampleTime=on
  Previous Time : Memory  InheritSampleTime=on
  Product : Product
  Product1 : Product
  Record : Record  FileSettingsInternal="{\"entries\":[{\"content\":{\"excelSettings\":{\"content\":{},\"type\":\"Streamout.ExcelSettings\"}},\"type\":\"Streamout.FileSettingStorage\",\"uuid\":\"\"}],\"packageUris\":[\"http:\\/\\/schema.mathworks.com\\/mf0\\/streamout_blocks\\/R2020a\"],\"version\":\"1.0\"}"  Layout=[1 1]  SignalsInternal="{\"entries\":[{\"content\":{\"signals\":[{\"content\":{\"blockPath\":[],\"dimensions\":[6,1],\"domain\":\"\",\"hasChildren\":true,\"lineColor\":\"#ff13a6\",\"port\":1,\"signalID\":3890,\"signalName\":\"MATLAB Function:2\"},\"type\":\"RecordBlkView.Signal\",\"uuid\":\"\"},{\"content\":{\"blockPath\":[],\"channel\":[1,1],\"dimensions\":[6,1],\"domain\":\"\",\"lineColor\":\"#77ac30\",\"parentID\":3890,\"plots\":[1],\"port\":1,\"signalID\":3891,\"signalName\":\"MAT ...(+1287 chars)"  VisualizationBindings="{\"sparklinesplugin\":{\"info\":[{\"bindingParametersList\":[],\"subplotID\":1}]}}"
  Record1 : Record  FileSettingsInternal="{\"entries\":[{\"content\":{\"excelSettings\":{\"content\":{},\"type\":\"Streamout.ExcelSettings\"}},\"type\":\"Streamout.FileSettingStorage\",\"uuid\":\"\"}],\"packageUris\":[\"http:\\/\\/schema.mathworks.com\\/mf0\\/streamout_blocks\\/R2020a\"],\"version\":\"1.0\"}"  Layout=[1 1]  SignalsInternal="{\"entries\":[{\"content\":{\"signals\":[{\"content\":{\"blockPath\":[],\"dimensions\":[6],\"domain\":\"\",\"hasChildren\":true,\"lineColor\":\"#22b573\",\"port\":1,\"signalID\":3878,\"signalName\":\"Eta 0-Order\"},\"type\":\"RecordBlkView.Signal\",\"uuid\":\"\"},{\"content\":{\"blockPath\":[],\"channel\":[1],\"dimensions\":[6],\"domain\":\"\",\"lineColor\":\"#0072bd\",\"parentID\":3878,\"port\":1,\"signalID\":3879,\"signalName\":\"Eta 0-Order\"},\"type\":\"Recor ...(+173 chars)"  VisualizationBindings="{\"sparklinesplugin\":{\"info\":[{\"bindingParametersList\":[],\"subplotID\":1}]}}"
  Record2 : Record  FileSettingsInternal="{\"entries\":[{\"content\":{\"excelSettings\":{\"content\":{},\"type\":\"Streamout.ExcelSettings\"}},\"type\":\"Streamout.FileSettingStorage\",\"uuid\":\"\"}],\"packageUris\":[\"http:\\/\\/schema.mathworks.com\\/mf0\\/streamout_blocks\\/R2020a\"],\"version\":\"1.0\"}"  Layout=[1 1]  SignalsInternal="{\"entries\":[{\"content\":{\"signals\":[{\"content\":{\"blockPath\":[],\"dimensions\":[1,6],\"domain\":\"\",\"hasChildren\":true,\"lineColor\":\"#d95319\",\"port\":1,\"signalID\":3861,\"signalName\":\"currentError\"},\"type\":\"RecordBlkView.Signal\",\"uuid\":\"\"},{\"content\":{\"blockPath\":[],\"channel\":[1,1],\"dimensions\":[1,6],\"domain\":\"\",\"lineColor\":\"#7e2f8e\",\"parentID\":3861,\"plots\":[1],\"port\":1,\"signalID\":3862,\"signalName\":\"currentE ...(+1252 chars)"  VisualizationBindings="{\"sparklinesplugin\":{\"info\":[{\"bindingParametersList\":[],\"subplotID\":1}]}}"
  Record3 : Record  FileSettingsInternal="{\"entries\":[{\"content\":{\"excelSettings\":{\"content\":{},\"type\":\"Streamout.ExcelSettings\"}},\"type\":\"Streamout.FileSettingStorage\",\"uuid\":\"\"}],\"packageUris\":[\"http:\\/\\/schema.mathworks.com\\/mf0\\/streamout_blocks\\/R2020a\"],\"version\":\"1.0\"}"  Layout=[1 1]  SignalsInternal="{\"entries\":[{\"content\":{\"signals\":[{\"content\":{\"blockPath\":[],\"dimensions\":[6,1],\"domain\":\"\",\"hasChildren\":true,\"lineColor\":\"#7e2f8e\",\"port\":1,\"signalID\":4102,\"signalName\":\"Product1\"},\"type\":\"RecordBlkView.Signal\",\"uuid\":\"\"},{\"content\":{\"blockPath\":[],\"channel\":[1,1],\"dimensions\":[6,1],\"domain\":\"\",\"lineColor\":\"#b746ff\",\"parentID\":4102,\"plots\":[1],\"port\":1,\"signalID\":4103,\"signalName\":\"Product1\"},\" ...(+1224 chars)"  VisualizationBindings="{\"sparklinesplugin\":{\"info\":[{\"bindingParametersList\":[],\"subplotID\":1}]}}"
  Record4 : Record  FileSettingsInternal="{\"entries\":[{\"content\":{\"excelSettings\":{\"content\":{},\"type\":\"Streamout.ExcelSettings\"}},\"type\":\"Streamout.FileSettingStorage\",\"uuid\":\"\"}],\"packageUris\":[\"http:\\/\\/schema.mathworks.com\\/mf0\\/streamout_blocks\\/R2020a\"],\"version\":\"1.0\"}"  Layout=[1 1]  SignalsInternal="{\"entries\":[{\"content\":{\"signals\":[{\"content\":{\"blockPath\":[],\"dimensions\":[6,1],\"domain\":\"\",\"hasChildren\":true,\"lineColor\":\"#4dbeee\",\"port\":1,\"signalID\":3844,\"signalName\":\"MATLAB Function:1\"},\"type\":\"RecordBlkView.Signal\",\"uuid\":\"\"},{\"content\":{\"blockPath\":[],\"channel\":[1,1],\"dimensions\":[6,1],\"domain\":\"\",\"lineColor\":\"#4dbeee\",\"parentID\":3844,\"plots\":[1],\"port\":1,\"signalID\":3845,\"signalName\":\"MAT ...(+1275 chars)"  VisualizationBindings="{\"sparklinesplugin\":{\"info\":[{\"bindingParametersList\":[],\"subplotID\":1}]}}"
  Record5 : Record  FileSettingsInternal="{\"entries\":[{\"content\":{\"excelSettings\":{\"content\":{},\"type\":\"Streamout.ExcelSettings\"}},\"type\":\"Streamout.FileSettingStorage\",\"uuid\":\"\"}],\"packageUris\":[\"http:\\/\\/schema.mathworks.com\\/mf0\\/streamout_blocks\\/R2020a\"],\"version\":\"1.0\"}"  Layout=[1 1]  SignalsInternal="{\"entries\":[{\"content\":{\"signals\":[{\"content\":{\"blockPath\":[],\"dimensions\":[1,6],\"domain\":\"\",\"hasChildren\":true,\"lineColor\":\"#139fff\",\"port\":1,\"signalID\":4136,\"signalName\":\"Sum1\"},\"type\":\"RecordBlkView.Signal\",\"uuid\":\"\"},{\"content\":{\"blockPath\":[],\"channel\":[1,1],\"dimensions\":[1,6],\"domain\":\"\",\"lineColor\":\"#ff13a6\",\"parentID\":4136,\"plots\":[1],\"port\":1,\"signalID\":4137,\"signalName\":\"Sum1\"},\"type\":\"R ...(+1184 chars)"  VisualizationBindings="{\"sparklinesplugin\":{\"info\":[{\"bindingParametersList\":[],\"subplotID\":1}]}}"
  Sum : Sum  Inputs=|++
  Sum1 : Sum  Inputs=|+++
  Switch : Switch  Criteria=u2 ~= 0  SaturateOnIntegerOverflow=off  InputSameDT=off
  "Sliding Mode Correction " : Outport
  wires:
  MATLAB Function/2(SSign) -> Record/1, Product/2
  currentErrorDot/1 -> MATLAB Function/3(currentErrorDot)
  currentError/1 -> MATLAB Function/2(currentError), Record2/1
  Product/1 -> Sum/2
  Product1/1 -> Record3/1, Sum/1
  MATLAB Function/1(SFlipTime) -> Record4/1, Product1/1, Previous S-Flip Time/1
  Sum/1 -> "Sliding Mode Correction "/1
  Previous S-Flip Time/1 -> MATLAB Function/1(PreviousSFlipTime)
  Eta 0-Order/1 -> Record1/1, Product/1
  Eta 1-Order/1 -> Product1/2
  lamda/1 -> MATLAB Function/4(lambda)
  Sum1/1 -> MATLAB Function/6(resetFlipTimeMask), Record5/1
  Set Point Changed/1 -> Sum1/1
  Motion Enabled/1 -> Invert Logic Signal/2
  Constant/1 -> Invert Logic Signal/1
  Constant1/1 -> Invert Logic Signal/3
  Previous Time/1 -> Switch/2, Switch/3, Delta T/2
  ros time/1 -> Previous Time/1, Delta T/1
  Switch/1 -> MATLAB Function/5(deltaTime)
  Delta T/1 -> Switch/1
  Have Gains Changed/1 -> Sum1/3
  Invert Logic Signal/1 -> Sum1/2

== matlab function SMC/Mathmatical Model/Calculate World 2 Body Rotm ==
function world2Body = fcn(currentWorldFramePosition)

%convert ros2 quat to matlab quat - quat is last 
quat = [currentWorldFramePosition(7), currentWorldFramePosition(4), currentWorldFramePosition(5), currentWorldFramePosition(6)];

%calculate the rotation matrix representing the current orientation
world2Body = quat2rotm(quat);

%matlab issue
world2Body = transpose(world2Body);

== matlab function SMC/Mathmatical Model/Fm/calculate body frame drag forces ==
function dragForces = fcn(currentBodyVelocities, dragCoefficents)

dragForces = zeros(6,1);

expectedDragCoefficentLength = 24;
if(expectedDragCoefficentLength ~= length(dragCoefficents))
    %drag coefficents are not the expected length
    return 
end

%reshape drag coefficents array into a more sensible form
dc = reshape(dragCoefficents, [expectedDragCoefficentLength / 6, 6]);

for i=1:6
    %calculate the forces created by drag
    dragForces(i) = dc(1, i) + abs(currentBodyVelocities(i)) * dc(2, i) + exp(abs(currentBodyVelocities(i)) / dc(4, i))* dc(3, i);

    %take into account sign
    sign = 0;
    if(currentBodyVelocities(i) ~= 0)
        sign = currentBodyVelocities(i) / abs(currentBodyVelocities(i));
    end

    dragForces(i) = sign * dragForces(i);
end

== matlab function SMC/MATLAB Function ==
function setPointChangedMask = fcn(previousSetPoint, newSetPoint)

setPointChangedMask = zeros(1,6);

%determine wether or not the set point has chnaged - element wise

previousEulerSetPoint = [previousSetPoint(1), previousSetPoint(2), previousSetPoint(3), quat2eul([previousSetPoint(7), previousSetPoint(4), previousSetPoint(5), previousSetPoint(6)])];
newEulerSetPoint = [newSetPoint(1), newSetPoint(2), newSetPoint(3), quat2eul([newSetPoint(7), newSetPoint(4), newSetPoint(5), newSetPoint(6)])];

%not changed = 0, true - everything else
setPointChangedMask = abs(previousEulerSetPoint - newEulerSetPoint);

%allow buffer on angular to account for slight shift due to conversion
%error...
for i=4:6
    if(setPointChangedMask(i) < .1)
        setPointChangedMask(i) = 0;
    end

    %catch nans and reset if they occur
    if(isnan(setPointChangedMask(i)))
        setPointChangedMask(i) = 1;
    end
end

== matlab function SMC/Mathmatical Model/S Block/MATLAB Function ==
function [SFlipTime, SSign] = fcn(PreviousSFlipTime, currentError, currentErrorDot, lambda, deltaTime, resetFlipTimeMask)

%FlipTime, SSign and Previous are 6 by arrays - 1 per dof

SFlipTime = PreviousSFlipTime;
SSign = zeros(6,1);

%calculate S
S = currentError + lambda' .* currentErrorDot';


%just so nothing explodes - ill be impressed if this happens
for i=1:6

    %ensure no S equals zero
    if(S(i) == 0)
        SSign(i) = 0;
    else
        SSign(i) = S(i) / abs(S(i));
    end
end


%see if Sdot has flipped
for i=1:6

    %if the flip time is not to be reset
    if(~resetFlipTimeMask(i))
        if(SFlipTime(i) * SSign(i) > 0)
            SFlipTime(i) = SFlipTime(i) + deltaTime * SSign(i);
        else
            SFlipTime(i) = deltaTime * SSign(i);
        end
    else
       SFlipTime(i) = 0;
    end
end

== matlab function SMC/Mathmatical Model/Normalize Error ==
function normalizedError = fcn(currentPosition, currentSetPoint)

normalized = zeros(1,6);

normalized(1) = currentPosition(1) - currentSetPoint(1);
normalized(2) = currentPosition(2) - currentSetPoint(2);
normalized(3) = currentPosition(3) - currentSetPoint(3);

W2B = [currentPosition(7), currentPosition(4), currentPosition(5), currentPosition(6)];
setQuat = [currentSetPoint(7), -currentSetPoint(4), -currentSetPoint(5), -currentSetPoint(6)];


%Talos Heading in Body Frame
Tbody = [1,0,0,0];

%Transform from Body 2 World
B2W = [W2B(1), -W2B(2), -W2B(3), -W2B(4)] / (norm(W2B) ^ 2);

%Talos Heading in World Frame
TWorld = quatmultiply(Tbody, B2W);

%Talos Heading in World Frame Conjugate
TWorldI = [TWorld(1), -TWorld(2), -TWorld(3), -TWorld(4)];

%Current Yaw Error
eQuat = quatmultiply(setQuat, TWorldI);

% %axis Error
axisError = [eQuat(2), eQuat(3), eQuat(4)];
if(eQuat(1) < 0)
    axisError = -axisError;
end


normalized(4) = axisError(1);
normalized(5) = axisError(2);
normalized(6) = axisError(3);

normalizedError = normalized;

== matlab function SMC/MATLAB Function1 ==
function haveGainsChangedMask = fcn(previousLamba, lamda, previousEta0, eta0, previousEta1, eta1)

%determine wether or not the set point has chnaged element wise
haveGainsChangedMask = abs(previousLamba - lamda) + abs(previousEta0 - eta0) + abs(previousEta1 - eta1);

== matlab function SMC/Mathmatical Model/Edot/Target Velocity Gravity Well ==
function targetVelocities = fcn(setPointError, controlParameters)

%the target velocities to converge to 
targetVelocities = zeros(6,1);

controlParametersExpectedLength = 12;
if(~length(controlParameters) == controlParametersExpectedLength)
    %params have not yet been assigned / assgined incorrectly
    return
end

controlParameters = reshape(controlParameters, [length(controlParameters) / 6, 6]);
%param(1,x) = max control value
%param(2,x) = the error where max control is reached

%velocity curves = param(1,x) * (-cos(error * pi / (2 * param(2,x)))^1/2 + 1)
for i=1:6
    if(controlParameters(2, i) == 0 || setPointError(i) == 0)
        targetVelocities(i) = 0;
    else
        %ensure the saturation error is not exceeded
        if(abs(setPointError(i)) > controlParameters(2, i))
            setPointError(i) = controlParameters(2, i) * setPointError(i) / abs(setPointError(i));
        end

        targetVelocities(i) = controlParameters(1,i) * (-cos(setPointError(i) * pi / (2 * controlParameters(2,i)))^(1/2) + 1);

        %enforce sign
        targetVelocities(i) = -(targetVelocities(i)) * setPointError(i) / abs(setPointError(i));
    end


end
